simulink model "testPSQ"  (R2016a)
settings: Solver=VariableStepAuto  StartTime=0.0  StopTime=10.0  RelTol=1e-3
undefined symbols (not defined in the file or in its folder): m, n
libraries: dspstat3 x1
settings Model: Creator=demo  LastModifiedBy=demo

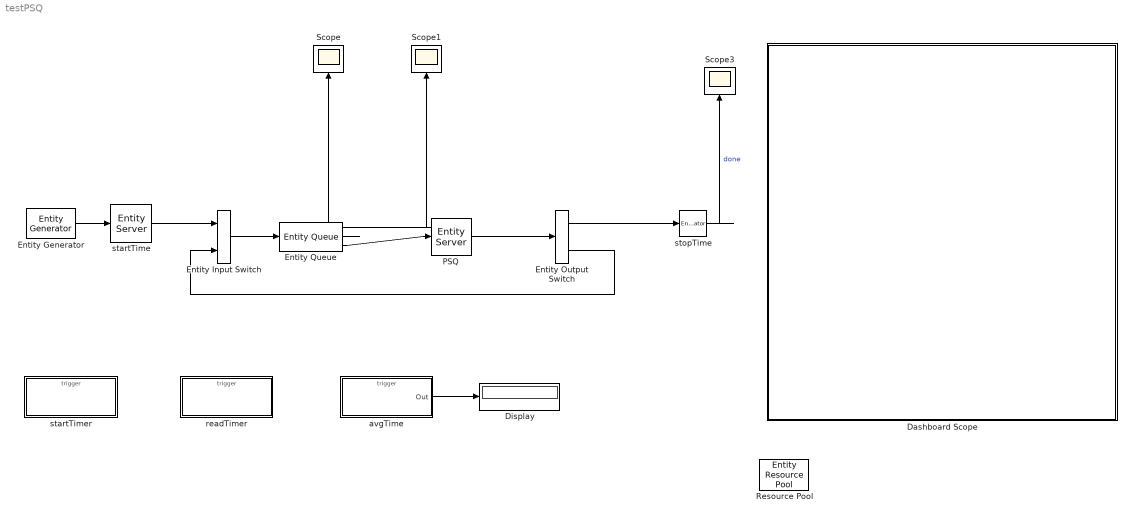
== system testPSQ ==
  Dashboard Scope : Subsystem  DialogController=hmiCreateDDGDialog  IsWebBlock=on  mask(MWDashboardBlock){webBlockId=93fdf2d6-6c09-4820-8f1f-cc3ef1f549fc, webBlockType=sdiscope, ShowInitialText=on, HMISrcModelName=testPSQ}
      mask prompts: webBlockId "WebBlock Id"; webBlockType "WebBlock Type"; HMISrcModelName "Source Model"
      mask Help: helpview([docroot '/mapfiles/simulink.map'], 'hmi_scope')
      mask Display:
      | if strcmp(get_param(bdroot(gcb),'BlockDiagramType'), 'library')
      |     image([(matlabroot) '/toolbox/simulink/hmi/icons/DashboardScope.png']);
      | end
  Display : Display
  Entity Input Switch : EntityInputSwitch  InputPortMessageModes=m,m  OutputPortMessageModes=m
  Entity Output Switch : EntityOutputSwitch  InputPortMessageModes=m  OutputPortMessageModes=m,m  SwitchingCriterion=From attribute  SwitchAttributeName=dest
  Entity Generator : EntityGenerator  OutputPortMessageModes=m  Period=2  AttributeName=ServiceTime|PreemptionPriority|timer|dest  AttributeInitialValue=10|1|0|1  EntityType=Structured  EntityTypeName=Entity
  Entity Queue : EntityQueue  InputPortMessageModes=m  OutputPortMessageModes=n,n,m  Capacity=inf  NumberEntitiesDeparted=on  NumberEntitiesInBlock=on
      settings: OutputPortMap=o0,o1,o5
  PSQ : EntityServer  InputPortMessageModes=m  OutputPortMessageModes=m  Capacity=1  ServiceTimeValue=.2  ServiceTimeAttributeName=PreemptionPriority  ServiceCompleteAction=|  WriteResidualTimeToAttribute=on  ResidualTimeAttributeName=PreemptionPriority
      | entity.ServiceTime = entity.ServiceTime - 1
      | 
      | if(entity.ServiceTime == 0)
      |     entity.dest = 1
      | else
      |     entity.dest = 2
  Resource Pool : EntityResourcePool
  Scope : Scope
  Scope1 : Scope
  Scope3 : Scope
  avgTime : Subsystem  TreatAsAtomicUnit=on
  readTimer : Subsystem  TreatAsAtomicUnit=on
  startTime : EntityServer  InputPortMessageModes=m  OutputPortMessageModes=m  Capacity=1  ServiceTimeValue=0  ServiceTimeAttributeName=PreemptionPriority  ServiceCompleteAction=entity.timer = startTimer();  WriteResidualTimeToAttribute=on  ResidualTimeAttributeName=PreemptionPriority
  startTimer : Subsystem  TreatAsAtomicUnit=on
  stopTime : EntityTerminator  InputPortMessageModes=m  EntryAction=|  NumberEntitiesArrived=on
      | % Read timer
      | elapsedTime = readTimer(entity.timer);
      | 
      | % Compute average
      | avgTime(elapsedTime);
      settings: OutputPortMap=o0
  wires:
  Entity Queue/2 -> Scope/1
  Entity Queue/1 -> Scope1/1
  Entity Queue/3 -> PSQ/1
  Entity Generator/1 -> startTime/1
  Entity Input Switch/1 -> Entity Queue/1
  PSQ/1 -> Entity Output Switch/1
  Entity Output Switch/1 -> stopTime/1
  Entity Output Switch/2 -> Entity Input Switch/2
  stopTime/1 -> Scope3/1  "done"
  startTime/1 -> Entity Input Switch/1
  avgTime/1(Out) -> Display/1

== system testPSQ/Dashboard Scope ==

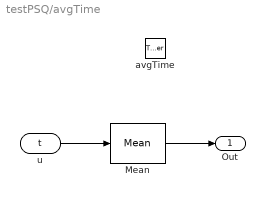
== system testPSQ/avgTime ==
  avgTime : TriggerPort  TriggerType=function-call  IsSimulinkFunction=on  FunctionName=avgTime  VariantControl=Variant
  Mean : dspstat3/Mean  run=off  reset_popup=None  InputProcessing=Columns as channels (frame based)  directionMode=Each column  dimension=1  roiEnable=off  roiType=Rectangles  roiPortion=Entire ROI  roiOutput=Individual statistics for each ROI  roiFlag=off  outputDataTypeStr=Inherit: Same as accumulator  outputLastDataTypeStr=Inherit: Same as accumulator  outputMin=[]  outputMax=[]  roundingMode=Floor  overflowMode=off
  u : ArgIn  DisableCoverage=on  ArgumentName=t
  Out : Outport
  wires:
  Mean/1 -> Out/1
  u/1 -> Mean/1

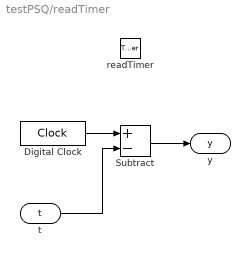
== system testPSQ/readTimer ==
  readTimer : TriggerPort  TriggerType=function-call  IsSimulinkFunction=on  FunctionName=readTimer  VariantControl=Variant
  Digital Clock : DigitalClock  SampleTime=-1
  Subtract : Sum  Inputs=+-
  t : ArgIn  DisableCoverage=on  ArgumentName=t
  y : ArgOut  DisableCoverage=on  ArgumentName=y
  wires:
  Digital Clock/1 -> Subtract/1
  Subtract/1 -> y/1
  t/1 -> Subtract/2

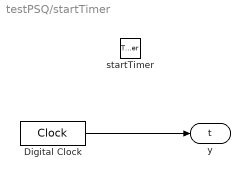
== system testPSQ/startTimer ==
  startTimer : TriggerPort  TriggerType=function-call  IsSimulinkFunction=on  FunctionName=startTimer  VariantControl=Variant
  Digital Clock : DigitalClock  SampleTime=-1
  y : ArgOut  DisableCoverage=on  ArgumentName=t
  wires:
  Digital Clock/1 -> y/1
